simulink model "experiment5"  (R2023a)
settings: Solver=VariableStepAuto  StartTime=0.0  StopTime=10.0  MaxStep=0.0001  RelTol=1e-4
settings Model: Creator=zou20  LastModifiedBy=zou20

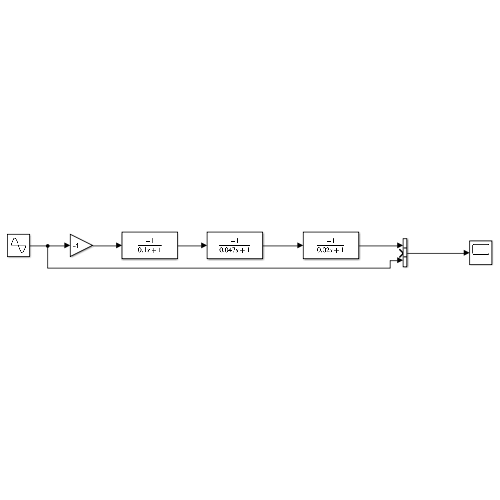
[thumbnail: Simulink's stored preview of the top-level diagram]
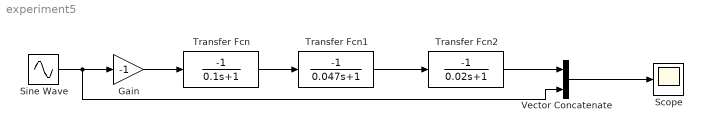
== system experiment5 ==
  Gain : Gain  Gain=-1
  Scope : Scope
  Sine Wave : Sin  SampleTime=0
  Transfer Fcn : TransferFcn  Numerator=[-1]  Denominator=[0.1 1]
  Transfer Fcn1 : TransferFcn  Numerator=[-1]  Denominator=[0.047 1]
  Transfer Fcn2 : TransferFcn  Numerator=[-1]  Denominator=[0.02 1]
  Vector Concatenate : Concatenate  NumInputs=3
  wires:
  Gain/1 -> Transfer Fcn/1
  Sine Wave/1 -> Gain/1, Vector Concatenate/3
  Transfer Fcn/1 -> Transfer Fcn1/1
  Transfer Fcn1/1 -> Transfer Fcn2/1
  Vector Concatenate/1 -> Scope/1
  Transfer Fcn2/1 -> Vector Concatenate/1
